simulink model "nonlin_quad_plant"  (R2024a)
settings: Solver=VariableStepAuto  StartTime=0.0  StopTime=300  FixedStep=sample_time  RelTol=1e-3
values from neighbouring files (symbols this model uses):
  drag_mat = [kdx 0 0; 0 kdy 0; 0 0 kdz]    [create_params.m]    (also in params.mat = [0.16481  0  0; 0  0.31892  0; 0  0  1.1e-06])
  g = 9.81    [create_params.m]    (also in params.mat)
  J = [inertia_xx; inertia_yy; inertia_zz]    [create_params.m]    (also in params.mat = [0.05 0.05 0.24])
  Jr = 8.54858e-06    [create_params.m]    (also in params.mat = 0.044)
  m = 0.68    [create_params.m]    (also in params.mat = 1.4)
settings Model: Creator=Lorenzo-Desk  LastModifiedBy=loca

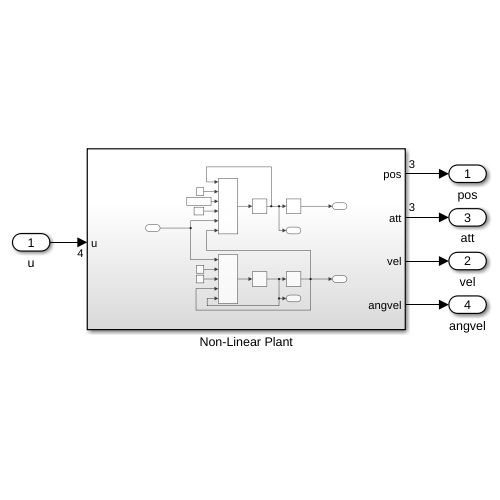
[thumbnail: Simulink's stored preview of the top-level diagram]
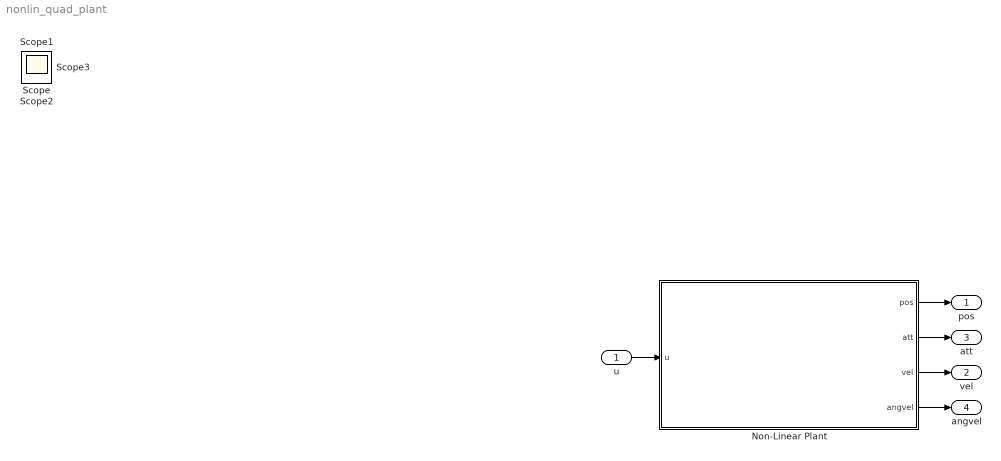
== system nonlin_quad_plant ==
  u : Inport
  Non-Linear Plant : Subsystem
  pos : Outport
  vel : Outport  Port=2
  att : Outport  Port=3
  angvel : Outport  Port=4
  Scope{,1..3} (4 alike) : Scope
  wires:
  u/1 -> Non-Linear Plant/1(u)
  Non-Linear Plant/1(pos) -> pos/1
  Non-Linear Plant/2(att) -> att/1
  Non-Linear Plant/3(vel) -> vel/1
  Non-Linear Plant/4(angvel) -> angvel/1

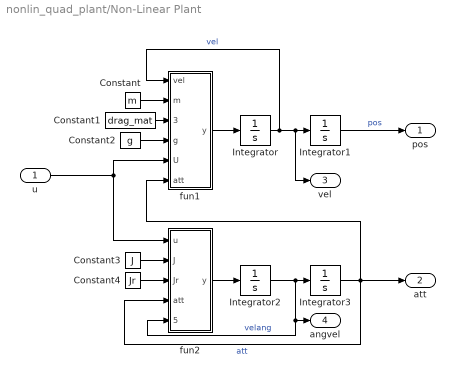
== system nonlin_quad_plant/Non-Linear Plant ==
  u : Inport  PortDimensions=4
  Constant : Constant  Value=m
  Constant1 : Constant  Value=drag_mat
  Constant2 : Constant  Value=g
  Constant3 : Constant  Value=J
  Constant4 : Constant  Value=Jr
  Integrator{,1..3} (4 alike) : Integrator
  fun1 : MATLAB Function  TreatAsAtomicUnit=on
  fun2 : MATLAB Function  TreatAsAtomicUnit=on
  pos : Outport  PortDimensions=3
  att : Outport  Port=2  PortDimensions=3
  vel : Outport  Port=3
  angvel : Outport  Port=4
  wires:
  u/1 -> fun2/1(u), fun1/5(U)
  Integrator2/1 -> angvel/1, fun2/5(velang), Integrator3/1  "velang"
  Constant4/1 -> fun2/3(Jr)
  fun1/1(y) -> Integrator/1
  Integrator/1 -> fun1/1(vel), vel/1, Integrator1/1  "vel"
  Constant/1 -> fun1/2(m)
  Integrator3/1 -> fun2/4(att), att/1, fun1/6(att)  "att"
  fun2/1(y) -> Integrator2/1
  Integrator1/1 -> pos/1  "pos"
  Constant1/1 -> fun1/3(drag_mat)
  Constant2/1 -> fun1/4(g)
  Constant3/1 -> fun2/2(J)

== matlab function nonlin_quad_plant/Non-Linear Plant/fun2 ==
  data: u input; y output; J input; Jr input; att input; velang input
function y = fcn(u, J, Jr, att, velang)
Jx = J(1); Jy = J(2); Jz = J(3);
phi = att(1); theta = att(2); psi = att(3);
phi_dot = velang(1); theta_dot = velang(2); psi_dot = velang(3);
Rr = [1 0 -sin(theta);
      0 cos(phi) sin(phi)*cos(theta);
      0 -sin(phi) cos(phi)*cos(theta)];
b_velang = inv(Rr)*velang;
B_phi_dot = velang(1); B_theta_dot = velang(2); B_psi_dot = velang(3);

y = zeros(3,1);
y(1) = (Jy-Jz/Jx)*B_theta_dot*B_psi_dot-Jr/Jx*B_theta_dot*u(1)+u(2)/Jx;
y(2) = (Jz-Jx/Jy)*B_phi_dot*B_psi_dot+Jr/Jy*B_phi_dot*u(1)+u(3)/Jy;
y(3) = (Jx-Jy/Jz)*B_phi_dot*B_theta_dot+u(4)/Jz;

%y(1) = (Jy-Jz/Jx)*theta_dot*psi_dot-Jr/Jx*theta_dot*u(1)+u(2)/Jx;
%y(2) = (Jz-Jx/Jy)*phi_dot*psi_dot+Jr/Jy*phi_dot*u(1)+u(3)/Jy;
%y(3) = (Jx-Jy/Jz)*phi_dot*theta_dot+u(4)/Jz;

== matlab function nonlin_quad_plant/Non-Linear Plant/fun1 ==
  data: vel input; m input; drag_mat input; g input; U input; att input; y output
function y = fcn(vel, m, drag_mat, g, U, att)
u = vel(1); v = vel(2); w = vel(3);
phi = att(1); theta = att(2); psi = att(3);
kdx = drag_mat(1,1); kdy = drag_mat(2,2); kdz = drag_mat(3,3);
y = zeros(3,1);
y(1) = -U(1)/m * (cos(phi)*sin(theta)*cos(psi) + sin(phi)*sin(psi)) - kdx*u/m;
y(2) = U(1)/m * (-cos(phi)*cos(theta)*sin(psi) + sin(phi) * cos(psi)) - kdy*v/m;
y(3) = -U(1)/m*cos(phi)*cos(theta) - kdz * w/m - g;
